simulink library "ssc"  (Simulink 8.1)
settings: Solver=ode1  StartTime=0.0  StopTime=Inf  FixedStep=0.001  RelTol=1e-3
PostLoadFcn:
  | , if any(exist('dsrtsu_mdlpostloadfcn', 'file') == [2, 3, 6]), try dsrtsu_mdlpostloadfcn('Execute', bdroot); catch fprintf('Error in PostLoadFcn (dsrtsu_mdlpostloadfcn) for model "%s":\n %s\n', bdroot, lasterr); end, end,
libraries: fmr x1
settings Model: DSRTSU_INTERNAL_RTI_VER=450  DSRTSU_INTERNAL_RTI_TYPE=rti1401  RTICANMMDATA=struct('GeneralSetupData',struct('modelroot','D:\ELN150201_TAIWAN\trunk\AdasDragon\software\sw_development\arch\app\acc','generalsettings',struct('filesettings',struct('destfolder',struct('Name','RTICANMM_FILES','Check',1),'buildfolder',struct('Name','.','Check',1),'AbsDestfolder',struct('Name','D:\ELN150201_TAIWAN\trunk\AdasDragon\software\sw_development\arch\app\acc\RTICANMM_FILES'),'AbsBuildfolder',struct('Name','D:\ELN150201_TAIWAN\trunk\AdasDragon\software\sw_development\arch\app\acc'))),'options',struct('addpaths',1,'rmpaths',1,'addtrcexclusion',logical(1),'cannavigator',struct('checkmonitoring',0),'show_usrtrc',0,'use_usrtrc',0),'advanced',struct('options',[1 1 1 1 1 1 1 1 1 1 1 1 1 1 1 1 1 1 1 1 1 1 1 1 1 1 1 1 1 1 1 1 1 1 1 1 1 1 1 1 1 1 1 1 1 1 1 1 1 1 1 1 1 1 1 1 1 1 1 1 1 1 1 1 1 1 1 1 1 1 1 1 1 1 1 1 1 1 1 1 1 1 1 1 1 1 1 1 1 1 1 1 1 1 1 1 1 1 1 1]),'MPSetup',{{}},'modelname','ssc','block','ssc'))  DSRTSU_INTERNAL_RTIFPGA=40  Creator=AT015555  LastModifiedBy=AT015555

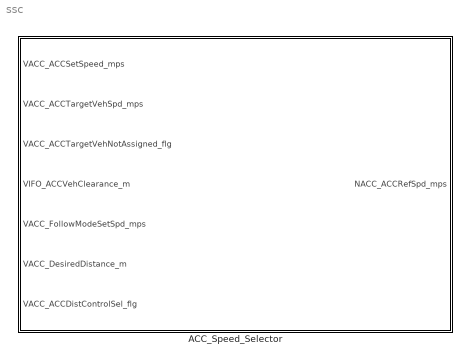
== system ssc ==
  ACC_Speed_Selector : Subsystem

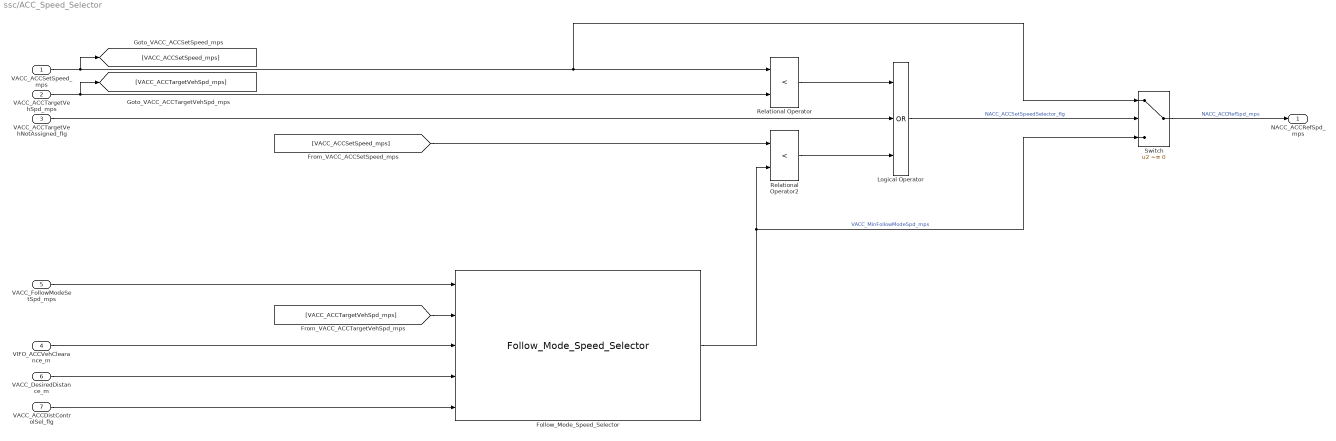
== system ssc/ACC_Speed_Selector ==
  VACC_ACCSetSpeed_mps : Inport
  VACC_ACCTargetVehSpd_mps : Inport  Port=2
  VACC_ACCTargetVehNotAssigned_flg : Inport  Port=3
  VIFO_ACCVehClearance_m : Inport  Port=4
  VACC_FollowModeSetSpd_mps : Inport  Port=5
  VACC_DesiredDistance_m : Inport  Port=6
  VACC_ACCDistControlSel_flg : Inport  Port=7
  Follow_Mode_Speed_Selector : fmr/Follow_Mode_Speed_Selector
  Logical Operator : Logic  Operator=OR  Inputs=3  AllPortsSameDT=off  OutDataTypeStr=boolean
  Relational Operator : RelationalOperator  Operator=<  OutDataTypeStr=boolean
  Relational Operator2 : RelationalOperator  Operator=<  OutDataTypeStr=boolean
  Switch : Switch  Criteria=u2 ~= 0
  NACC_ACCRefSpd_mps : Outport
  wires:
  [VACC_ACCSetSpeed_mps] -> Relational Operator2/1
  VACC_ACCSetSpeed_mps/1 -> [VACC_ACCSetSpeed_mps], Relational Operator/1, Switch/1
  Relational Operator2/1 -> Logical Operator/3
  VACC_ACCTargetVehSpd_mps/1 -> Relational Operator/2, [VACC_ACCTargetVehSpd_mps]
  Relational Operator/1 -> Logical Operator/1
  Logical Operator/1 -> Switch/2  "NACC_ACCSetSpeedSelector_flg"
  VACC_ACCTargetVehNotAssigned_flg/1 -> Logical Operator/2
  Switch/1 -> NACC_ACCRefSpd_mps/1  "NACC_ACCRefSpd_mps"
  Follow_Mode_Speed_Selector/1 -> Switch/3, Relational Operator2/2  "VACC_MinFollowModeSpd_mps"
  VACC_FollowModeSetSpd_mps/1 -> Follow_Mode_Speed_Selector/1
  [VACC_ACCTargetVehSpd_mps] -> Follow_Mode_Speed_Selector/2
  VIFO_ACCVehClearance_m/1 -> Follow_Mode_Speed_Selector/3
  VACC_DesiredDistance_m/1 -> Follow_Mode_Speed_Selector/4
  VACC_ACCDistControlSel_flg/1 -> Follow_Mode_Speed_Selector/5
